simulink model "LAB5T2"  (R2018b)
settings: Solver=VariableStepAuto  StartTime=0.0  StopTime=1000  RelTol=1e-3
settings Model: Creator=aloisia  LastModifiedBy=aloisia

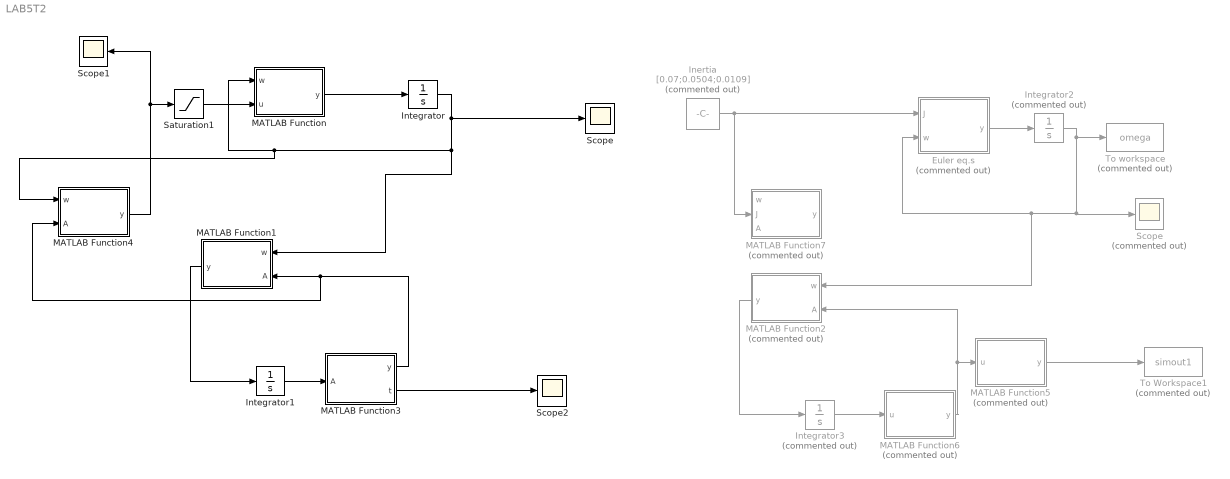
== system LAB5T2 ==
  Euler eq.s : MATLAB Function  Commented=on  TreatAsAtomicUnit=on
  Inertia : Constant  Commented=on  Value=[0.07;0.0504;0.0109]
  Integrator : Integrator  InitialCondition=[0.1; 0.1; 0.1]
  Integrator1 : Integrator  InitialCondition=[-0.782 0 -0.6233;-0.6233 0 -0.782;0 -1 0]
  Integrator2 : Integrator  Commented=on  InitialCondition=[0.45; 0.52; 0.55]
  Integrator3 : Integrator  Commented=on  InitialCondition=[1 0 0;0 1 0;0 0 1]
  MATLAB Function : MATLAB Function  TreatAsAtomicUnit=on
  MATLAB Function1 : MATLAB Function  TreatAsAtomicUnit=on
  MATLAB Function2 : MATLAB Function  Commented=on  TreatAsAtomicUnit=on
  MATLAB Function3 : MATLAB Function  TreatAsAtomicUnit=on
  MATLAB Function4 : MATLAB Function  TreatAsAtomicUnit=on
  MATLAB Function5 : MATLAB Function  Commented=on  TreatAsAtomicUnit=on
  MATLAB Function6 : MATLAB Function  Commented=on  TreatAsAtomicUnit=on
  MATLAB Function7 : MATLAB Function  Commented=on  TreatAsAtomicUnit=on
  Saturation1 : Saturate  UpperLimit=1e-3  LowerLimit=-1e-3  ZeroCross=off
  Scope : Scope
  "Scope " : Scope  Commented=on
  Scope1 : Scope
  Scope2 : Scope
  To Workspace1 : ToWorkspace  Commented=on  VariableName=simout1  SaveFormat=Timeseries  SampleTime=-1
  To workspace : ToWorkspace  Commented=on  VariableName=omega  SampleTime=-1
  wires:
  MATLAB Function3/1(y) -> MATLAB Function4/2(A), MATLAB Function1/2(A)
  MATLAB Function/1(y) -> Integrator/1
  Integrator1/1 -> MATLAB Function3/1(A)
  Integrator/1 -> MATLAB Function4/1(w), MATLAB Function/1(w), MATLAB Function1/1(w), Scope/1
  MATLAB Function1/1(y) -> Integrator1/1
  MATLAB Function4/1(y) -> Scope1/1, Saturation1/1
  Saturation1/1 -> MATLAB Function/2(u)
  Euler eq.s/1(y) -> Integrator2/1
  Inertia/1 -> MATLAB Function7/2(J), Euler eq.s/1(J)
  Integrator2/1 -> To workspace/1, MATLAB Function2/1(w), Euler eq.s/2(w), "Scope "/1
  MATLAB Function6/1(y) -> MATLAB Function5/1(u), MATLAB Function2/2(A)
  Integrator3/1 -> MATLAB Function6/1(u)
  MATLAB Function5/1(y) -> To Workspace1/1
  MATLAB Function2/1(y) -> Integrator3/1
  MATLAB Function3/2(t) -> Scope2/1

== matlab function LAB5T2/MATLAB Function1 ==
  data: w input; y output; A input
function y = Kinematic(w,A)

W=[0 -w(3) w(2);w(2) 0 -w(1);-w(2) w(1) 0];
Adot=-W*A;
y=Adot;
end

== matlab function LAB5T2/MATLAB Function ==
  data: w input; u input; y output
function y = Euler(w,u)
%First laboratory

%Datas
J1=0.01;
J2=0.05;
J3=0.07;

omx=w(1);
omy=w(2);
omz=w(3);

%Formula
omxdot=(J2-J3)/J1*omy*omz + u(1)/J1;
omydot=(J3-J1)/J2*omx*omz + u(2)/J2;
omzdot=(J1-J2)/J3*omy*omx + u(3)/J3;

y=[omxdot; omydot; omzdot];

end

== matlab function LAB5T2/Euler eq.s ==
  data: J input; w input; y output
function y = euler_eqs(J,w)

J1=J(1);
J2=J(2);
J3=J(3);

w_dot = zeros(3,1);

c1 = ((J2-J3)/J1);
c2 = ((J3-J1)/J2);
c3 = ((J1-J2)/J3);

w_dot(1) = c1*w(2)*w(3) + w(1)/J1;
w_dot(2) = c2*w(1)*w(3) + w(2)/J2;
w_dot(3) = c3*w(2)*w(1) + w(3)/J3;

y=w_dot;

== matlab function LAB5T2/MATLAB Function3 ==
  data: A input; y output; t output
function [y , t] = Orthonorm(A)

t=abs(trace(eye(3)-A'*A));
% tt = [];
% k = 0;
% while k<1000
%         A=(1.5)*u-u*u'*0.5*u;
%         t=abs(trace(eye(3)-A'*A));
%         u=A;
%         k = k+1;
% end
    while t>0.00000000000000001 
        A=(1.5)*A-A*A'*0.5*A;
        t=abs(trace(eye(3)-A'*A));
        
    end
% 
y=A;
t=t;
end

== matlab function LAB5T2/MATLAB Function4 ==
  data: w input; A input; y output
function y = control_law(w,A)

J1=0.01;
J2=0.05;
J3=0.07;

J = diag([J1,J2,J3]);

% Set k1 and k2 due to have a faster stabilization
k1 = 0.9;
k2 = 0.9;

K = k1 * J;
C = k2 * J;

% Set control matrix Ac
Ac = eye(3);
% Set error matrix Ae
Ae = A*(Ac');
d = (Ae' - Ae);
e = [d(3,2);d(1,3);d(2,1)];

u = - K*e - C*w;

y=u;

== matlab function LAB5T2/MATLAB Function2 ==
  data: w input; y output; A input
function y = fcn(w,A)

W=[0 -w(3) w(2);w(2) 0 -w(1);-w(2) w(1) 0];
Adot=-W*A;
y=Adot;
end

== matlab function LAB5T2/MATLAB Function5 ==
  data: u input; y output
function y = fcn(u)

t=trace(eye(3)-(u')*u);
y=t;

end

== matlab function LAB5T2/MATLAB Function6 ==
  data: u input; y output
function y = fcn(u)

t=abs(trace(eye(3)-u'*u));
while t>0.00000001
    A=(1.5)*u-u*u'*0.5*u;
    t=abs(trace(eye(3)-A'*A));
    u=A;
end

y=u;
end

== matlab function LAB5T2/MATLAB Function7 ==
  data: w input; J input; y output; A input
function y = fcn(w,J,A)


end
